simulink library "Input_Water_Glycol"  (Simulink 8.2)
settings: Solver=ode45  StartTime=0.0  StopTime=10.0  RelTol=1e-3
settings Model: Creator=lena.frank  LastModifiedBy=drhf

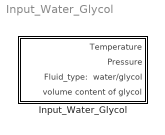
== system Input_Water_Glycol ==
  Input_Water_Glycol : Subsystem  mask(input_water_glycol){T=20, p=1e5, g=0.4}
      mask prompts: T "temperature (scalar or vector) [°C]"; p "pressure [Pa]"; g "volume content of glycol [0..1]"
      mask help: Sets all values for the water - propylen-glycol mixtures.
      mask Help: web(fullfile(path_carnot('help'),'input_material.html'),'-helpbrowser')

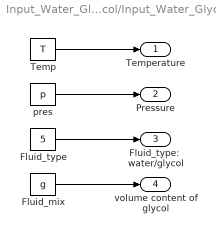
== system Input_Water_Glycol/Input_Water_Glycol ==
  Fluid_mix : Constant  Value=g
  Fluid_type : Constant  Value=5
  Temp : Constant  Value=T
  pres : Constant  Value=p
  Temperature : Outport
  Pressure : Outport  Port=2
  Fluid_type:  water/glycol : Outport  Port=3
  "volume content of glycol " : Outport  Port=4
  wires:
  Fluid_mix/1 -> "volume content of glycol "/1
  Fluid_type/1 -> Fluid_type:  water/glycol/1
  Temp/1 -> Temperature/1
  pres/1 -> Pressure/1
